simulink model "csc_sc_wsim_stored_command_hrn"  (R2014b)
settings: Solver=FixedStepDiscrete  StartTime=0.0  StopTime=100  FixedStep=0.01  RelTol=1e-3
libraries: csc_sc_wsim_stored_command_lib x1, csu_sch_scheduler_lib x1
settings Model: Creator=escrane  LastModifiedBy=mstewart
settings DebuggingCC: UnderspecifiedInitializationDetection=Classic  MergeDetectMultiDrivingBlocksExec=none  StateNameClashWarn=warning

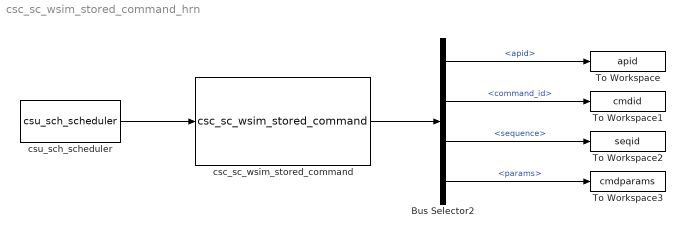
== system csc_sc_wsim_stored_command_hrn ==
  Bus Selector2 : BusSelector  OutputSignals=apid,command_id,sequence,params
  To Workspace : ToWorkspace  VariableName=apid  SaveFormat=Timeseries  SampleTime=-1
  To Workspace1 : ToWorkspace  VariableName=cmdid  SaveFormat=Timeseries  SampleTime=-1
  To Workspace2 : ToWorkspace  VariableName=seqid  SaveFormat=Timeseries  SampleTime=-1
  To Workspace3 : ToWorkspace  VariableName=cmdparams  SaveFormat=Timeseries  SampleTime=-1
  csc_sc_wsim_stored_command : csc_sc_wsim_stored_command_lib/csc_sc_wsim_stored_command  Tag=OFSW
  csu_sch_scheduler : csu_sch_scheduler_lib/csu_sch_scheduler
  wires:
  csu_sch_scheduler/1 -> csc_sc_wsim_stored_command/1
  Bus Selector2/1 -> To Workspace/1  "<apid>"
  Bus Selector2/2 -> To Workspace1/1  "<command_id>"
  Bus Selector2/3 -> To Workspace2/1  "<sequence>"
  Bus Selector2/4 -> To Workspace3/1  "<params>"
  csc_sc_wsim_stored_command/1 -> Bus Selector2/1
